simulink model "vor"  (R2023b)
settings: Solver=FixedStepDiscrete  StartTime=0.0  StopTime=0.1  FixedStep=1/(2*108200000)  RelTol=1e-3
model workspace (MAT data in the model file):
  theta = 0
undefined symbols (not defined in the file or in its folder): dfilt
libraries: dsparch4 x3
settings Model: Creator=86134  LastModifiedBy=86134

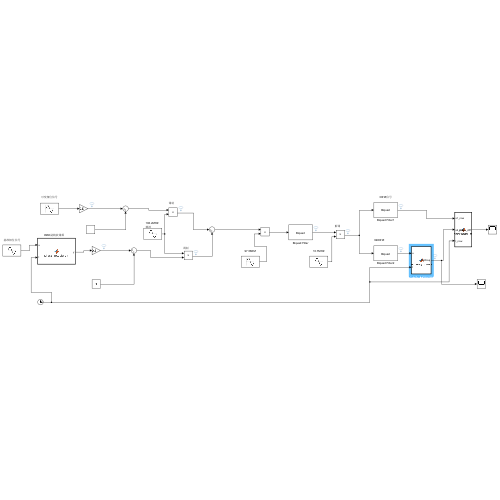
[thumbnail: Simulink's stored preview of the top-level diagram]
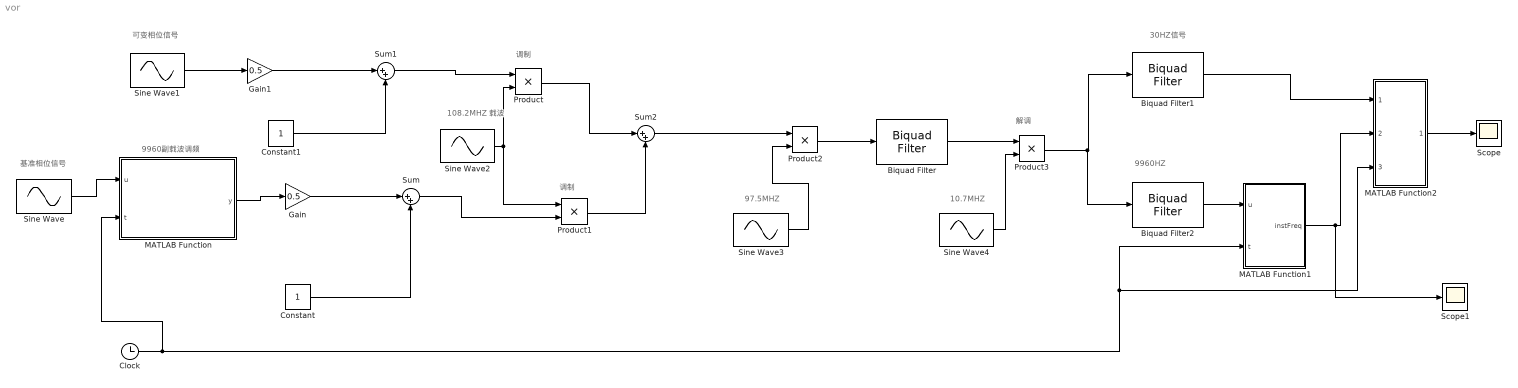
== system vor ==
  note: 9960HZ
  note: 30HZ信号
  note: 解调
  note: 10.7MHZ
  note: 97.5MHZ
  note: 调制
  note: 调制
  note: 9960副载波调频
  note: 可变相位信号
  note: 基准相位信号
  note: 108.2MHZ
      | 载波
  Biquad Filter : dsparch4/Biquad Filter  FilterSource=Dialog parameters  CoeffSource=Specify via dialog  FilterObject=dfilt.df2tsos([1 0.3 0.4],[1 0.1 0.2])  IIRFiltStruct=Direct form II transposed  BiQuadCoeffs=[0.000309679259585553 0 -0.000309679259585553 1 -1.9039833259881 0.9999117719419;0.000309679259585553 0 -0.000309679259585553 1 -1.90435830946092 0.99991194025141;0.000309653073416402 0 -0.000309653073416402 1 -1.9038373878921 0.99974250523878;0.000309653073416402 0 -0.000309653073416402 1 -1.90418224582671 0.999742956639612;0.00030963011966402 0 -0.00030963011966402 1 -1.90372534969385 0.999594175237536;0.00030963011966402 0 -0.00030963011966402 1 -1.90401205253472 0.999594766355106;0.000309612255205228 0 -0.000309612255205228 1 -1.90365627998478 0.99947880361806;0.000309612255205228 0 -0.000309612255205228 1 -1.90386148144516 0.999479346782633;0.000309600924376546 0 -0.000309600924376546 1 -1.90363574550684 0.999405718787672;0.000309600924376546 0 -0.000309600924376546 1 -1.90374271167913 0.999406041570626;0.000309597042893794 0 -0.000309597042893794 1 -1.90366536918465 0.999380805914212]  ScaleValues=1  IC=0  ICnum=0  ICden=0  a0Flag=Warning  optimizeScaleValues=on  ScaleValueMode=Specify via input port (g)  roundingMode=Floor  overflowMode=off  scaleValueFracLength=14  denProdOutputFracLength=30  denAccumFracLength=30  secondMemoryFracLength=15
      settings: LibrarySourceBlock=dsphdlsupportfiltering/Biquad Filter
  Biquad Filter1 : dsparch4/Biquad Filter  FilterSource=Dialog parameters  CoeffSource=Specify via dialog  FilterObject=dfilt.df2tsos([1 0.3 0.4],[1 0.1 0.2])  IIRFiltStruct=Direct form II transposed  BiQuadCoeffs=[8.25050886782997e-13 1.65010177356599e-12 8.25050886782997e-13 1 -1.99999969996181 0.999999699965108;8.25050642615194e-13 1.65010128523039e-12 8.25050642615194e-13 1 -1.99999910807646 0.999999108079758;8.25050408483965e-13 1.65010081696793e-12 8.25050408483965e-13 1 -1.99999854052069 0.999998540523993;8.25050190775778e-13 1.65010038155156e-12 8.25050190775778e-13 1 -1.9999980127759 0.9999980127792;8.25049995429113e-13 1.65009999085823e-12 8.25049995429113e-13 1 -1.99999753923751 0.999997539240807;8.25049827772484e-13 1.65009965554497e-12 8.25049827772484e-13 1 -1.99999713282232 0.999997132825623;8.2504969237909e-13 1.65009938475818e-12 8.2504969237909e-13 1 -1.99999680461621 0.999996804619506;8.25049592942076e-13 1.65009918588415e-12 8.25049592942076e-13 1 -1.99999656357168 0.999996563574982;8.25049532173798e-13 1.6500990643476e-12 8.25049532173798e-13 1 -1.99999641626375 0.999996416267054;9.08322361131686e-07 9.08322361131686e-07 0 1 -0.999998183355278 0]  ScaleValues=1  IC=0  ICnum=0  ICden=0  a0Flag=Warning  optimizeScaleValues=on  ScaleValueMode=Specify via input port (g)  roundingMode=Floor  overflowMode=off  scaleValueFracLength=14  denProdOutputFracLength=30  denAccumFracLength=30  secondMemoryFracLength=15
      settings: LibrarySourceBlock=dsphdlsupportfiltering/Biquad Filter
  Biquad Filter2 : dsparch4/Biquad Filter  FilterSource=Dialog parameters  CoeffSource=Specify via dialog  FilterObject=dfilt.df2tsos([1 0.3 0.4],[1 0.1 0.2])  IIRFiltStruct=Direct form II transposed  BiQuadCoeffs=[1.54972826459198e-05 0 -1.54972826459198e-05 1 -1.99999631052065 0.999996406775232;1.54972826459198e-05 0 -1.54972826459198e-05 1 -1.99999658111131 0.999996652644253;1.54972302145863e-05 0 -1.54972302145863e-05 1 -2.00014455650503 1.00014465153035;1.54972302145863e-05 0 -1.54972302145863e-05 1 -1.99983480215815 0.999834898813958;1.54971817612215e-05 0 -1.54971817612215e-05 1 -2.00001038465217 1.00001046835646;1.54971817612215e-05 0 -1.54971817612215e-05 1 -1.99995646783013 0.999956552379112;1.54971397153356e-05 0 -1.54971397153356e-05 1 -1.9999777969562 0.999977912082565;1.54971397153356e-05 0 -1.54971397153356e-05 1 -1.9999782031958 0.99997825538714;1.54971061851057e-05 0 -1.54971061851057e-05 1 -2.0001028480177 1.0001029381946;1.54971061851057e-05 0 -1.54971061851057e-05 1 -1.9998444977741 0.999844591392313;1.54970828516985e-05 0 -1.54970828516985e-05 1 -1.99997061266138 0.999970714363168;1.54970828516985e-05 0 -1.54970828516985e-05 1 -1.99997071064441 0.999970775884151;1.54970708850048e-05 0 -1.54970708850048e-05 1 -1.99996904345403 0.999969140589439;1.54970708850048e-05 0 -1.54970708850048e-05 1 -1.9999691911831 0.999969260896345]  ScaleValues=1  IC=0  ICnum=0  ICden=0  a0Flag=Warning  optimizeScaleValues=on  ScaleValueMode=Specify via input port (g)  roundingMode=Floor  overflowMode=off  scaleValueFracLength=14  denProdOutputFracLength=30  denAccumFracLength=30  secondMemoryFracLength=15
      settings: LibrarySourceBlock=dsphdlsupportfiltering/Biquad Filter
  Clock : Clock
  Constant : Constant
  Constant1 : Constant
  Gain : Gain  Gain=0.5
  Gain1 : Gain  Gain=0.5
  MATLAB Function : MATLAB Function  TreatAsAtomicUnit=on
  MATLAB Function1 : MATLAB Function  TreatAsAtomicUnit=on
  MATLAB Function2 : MATLAB Function  TreatAsAtomicUnit=on
  Product{,1..3} (4 alike) : Product
  Scope : Scope
  Scope1 : Scope
  Sine Wave : Sin  Frequency=30*2*pi  SampleTime=0
  Sine Wave1 : Sin  Frequency=30*2*pi  Phase=theta  SampleTime=0
  Sine Wave2 : Sin  Frequency=108200000*2*pi  SampleTime=0
  Sine Wave3 : Sin  Frequency=97500000*2*pi  SampleTime=0
  Sine Wave4 : Sin  Frequency=10700000*2*pi  SampleTime=0
  Sum : Sum  Inputs=|++
  Sum1 : Sum  Inputs=|++
  Sum2 : Sum  Inputs=|++
  wires:
  Sine Wave/1 -> MATLAB Function/1(u)
  MATLAB Function/1(y) -> Gain/1
  Gain/1 -> Sum/1
  Constant/1 -> Sum/2
  Sine Wave1/1 -> Gain1/1
  Gain1/1 -> Sum1/1
  Constant1/1 -> Sum1/2
  Sum1/1 -> Product/1
  Sine Wave2/1 -> Product1/1, Product/2
  Sum/1 -> Product1/2
  Product/1 -> Sum2/1
  Product1/1 -> Sum2/2
  Sum2/1 -> Product2/1
  Sine Wave3/1 -> Product2/2
  Product2/1 -> Biquad Filter/1
  Biquad Filter/1 -> Product3/1
  Sine Wave4/1 -> Product3/2
  Product3/1 -> Biquad Filter2/1, Biquad Filter1/1
  Biquad Filter2/1 -> MATLAB Function1/1(u)
  Biquad Filter1/1 -> MATLAB Function2/1(s1_now)
  MATLAB Function1/1(instFreq) -> Scope1/1, MATLAB Function2/2(s2_now)
  MATLAB Function2/1(phase_diff) -> Scope/1
  Clock/1 -> MATLAB Function/2(t), MATLAB Function2/3(t_now), MATLAB Function1/2(t)

== matlab function vor/MATLAB Function1 ==
  data: u input; instFreq output; t input
function instFreq = frequency_demod(u, t)
% u: 输入信号
% t: 当前时间
% fc: 载波频率 (9960 Hz)
% fs: 采样频率 (1/固定步长)
fc=9960;
fs=2*108200000;
% 初始化持久变量
persistent last_phase last_unwrapped_phase last_I last_Q;
if isempty(last_phase)
    last_phase = 0;
    last_unwrapped_phase = 0;
    last_I = 0;
    last_Q = 0;
end
% 1. 正交下变频
I = u * cos(2*pi*fc*t);  % 同相分量
Q = u * sin(2*pi*fc*t);  % 正交分量
% 2. 一阶低通滤波 (截止频率≈500Hz)
alpha = 2*pi*500/fs;  % 滤波系数
I_filt = (1-alpha)*last_I + alpha*I;
Q_filt = (1-alpha)*last_Q + alpha*Q;
% 3. 计算相位
phase = atan2(Q_filt, I_filt);
% 4. 相位解卷绕
delta = phase - last_phase;
delta_adjusted = mod(delta + pi, 2*pi) - pi;
unwrapped_phase = last_unwrapped_phase + delta_adjusted;
% 5. 计算瞬时频率
instFreq = fc + (unwrapped_phase - last_unwrapped_phase) * fs/(2*pi);
% 更新持久变量
last_phase = phase;
last_unwrapped_phase = unwrapped_phase;
last_I = I_filt;
last_Q = Q_filt;
end

== matlab function vor/MATLAB Function ==
  data: u input; y output; t input
function y = phase_modulation(u,t)
    % u: 输入的正弦信号
    % fc: 载波频率 (Hz)
    % fs: 系统采样频率 (Hz)
    % kp: 相位调制指数
    fc=9960;
    fs=2*108200000;
    kp=16;

    % 计算相位调制
    phase = 2 * pi * fc * t + kp * u;
    y = cos(phase);
end

== matlab function vor/MATLAB Function2 ==
  data: s1_now input; s2_now input; t_now input; phase_diff output
function phase_diff = calcPhaseDiff( s1_now, s2_now,t_now)
f=30;
% 声明持久变量以保存状态
persistent prev_s1 prev_s2 prev_t
persistent t_last_z1 t_last_z2 last_phase_diff
persistent initialized T
% 初始化变量
if isempty(initialized)
    % 第一次调用函数时初始化
    prev_s1 = 0;
    prev_s2 = 0;
    prev_t = t_now;
    t_last_z1 = NaN;
    t_last_z2 = NaN;
    last_phase_diff = NaN;
    T = 1/f;  % 信号周期
    initialized = true;
end
% 计算时间步长
dt = t_now - prev_t;
% 检测信号1的上升沿过零点 (从负到正)
if (prev_s1 <= 0 && s1_now > 0)
    % 使用线性插值精确计算过零点时间
    if dt > 0  % 避免除以零
        interp_factor = -prev_s1 / (s1_now - prev_s1);
        t_z1 = prev_t + interp_factor * dt;
        t_last_z1 = t_z1;
    end
end
% 检测信号2的上升沿过零点 (从负到正)
if (prev_s2 <= 0 && s2_now > 0)
    % 使用线性插值精确计算过零点时间
    if dt > 0  % 避免除以零
        interp_factor = -prev_s2 / (s2_now - prev_s2);
        t_z2 = prev_t + interp_factor * dt;
        t_last_z2 = t_z2;
    end
end

% 当两个信号都有有效的过零点时计算相位差
if ~isnan(t_last_z1) && ~isnan(t_last_z2)
    % 计算时间差
    delta_t = t_last_z1 - t_last_z2;
    
    % 归一化时间差到[-T/2, T/2]范围
    if delta_t > T/2
        delta_t = delta_t - T;
    elseif delta_t < -T/2
        delta_t = delta_t + T;
    end
    
    % 计算相位差 (角度)
    phase_diff_deg = (delta_t / T) * 360;
    
    % 确保相位差在 [-180, 180] 范围内
    if phase_diff_deg > 180
        phase_diff_deg = phase_diff_deg - 360;
    elseif phase_diff_deg < -180
        phase_diff_deg = phase_diff_deg + 360;
    end
    
    last_phase_diff = phase_diff_deg;
end
% 更新状态变量
prev_s1 = s1_now;
prev_s2 = s2_now;
prev_t = t_now;

% 设置输出
if ~isnan(last_phase_diff)
    phase_diff = last_phase_diff;
else
    % 如果还没有计算出相位差，返回0（或NaN，根据需求）
    phase_diff = 0;
end
end
